simulink model "final"  (R2023b)
settings: Solver=FixedStepAuto  StartTime=0.0  StopTime=60  RelTol=1e-3
undefined symbols (not defined in the file or in its folder): DiscIntNeverNeededParam
libraries: arduinolib x16, simulink x12, mobileRoboticsTrainingLib x1
settings Model: ExtModeTrigDuration=2  Creator=cameronclark  LastModifiedBy=cameronclark
settings OptimizationCC: EnhancedBackFolding=on  PassReuseOutputArgsAs=Individual arguments  ZeroExternalMemoryAtStartup=off  ZeroInternalMemoryAtStartup=off  MaxStackSize=64  OptimizeBlockOrder=speed  DifferentSizesBufferReuse=on  OptimizationCustomize=off  EfficientTunableParamExpr=on
settings DebuggingCC: ParameterTunabilityLossMsg=error
settings HardwareCC: ProdBitPerPointer=32  ProdBitPerSizeT=32  ProdBitPerPtrDiffT=32  ProdLargestAtomicInteger=Long  ProdLargestAtomicFloat=Double  ProdWordSize=32  ProdHWDeviceType=ARM Compatible->ARM Cortex  UseEmbeddedCoderFeatures=off  UseSimulinkCoderFeatures=off
settings SFSimCC: MATLABDynamicMemAlloc=off
settings RTWCC: Description=Embedded Coder  SystemTargetFile=ert.tlc  HardwareBoard=Arduino Nano 33 IoT  TemplateMakefile=ert_default_tmf  Toolchain=Arduino ARM  BuildConfiguration=Faster Runs
settings CodeAppCC: ForceParamTrailComments=on  IgnoreCustomStorageClasses=off  OperatorAnnotations=on  SimulinkDataObjDesc=on  SFDataObjDesc=on  InsertBlockDesc=on
settings ERTTargetCC: SupportContinuousTime=on  SupportNonInlinedSFcns=on  SupportVariableSizeSignals=on  ExtModeTransport=3  ExtModeStaticAlloc=on  ExtModeAutomaticAllocSize=off  ExtModeStaticAllocSize=8192  ExtModeMexFile=ext_xcp  ExtModeIntrfLevel=Level2 - Open

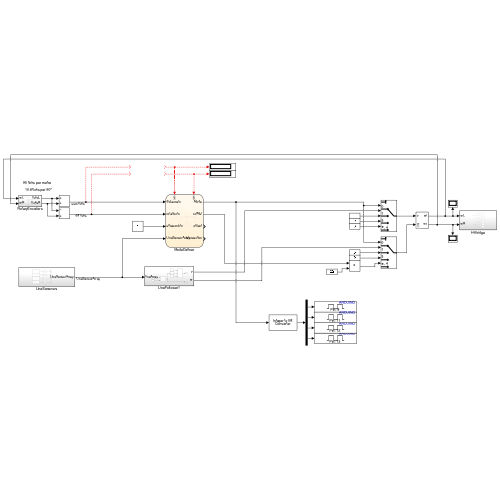
[thumbnail: Simulink's stored preview of the top-level diagram]
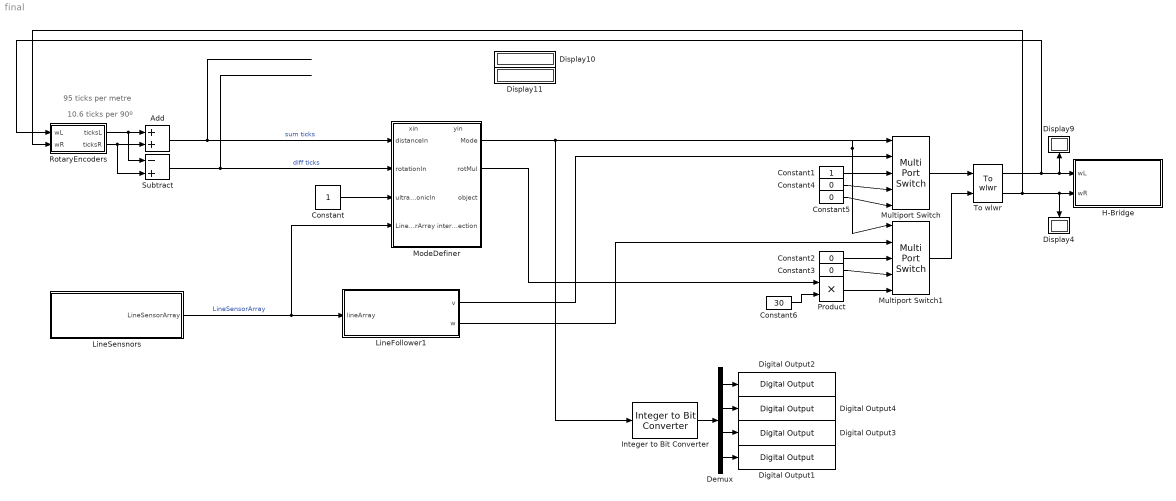
== system final ==
  note: 95 ticks per metre
  note: 10.6 ticks per 90º
  Add : Sum
  Constant : Constant
  Constant1 : Constant
  Constant{2..5} (4 alike) : Constant  Value=0
  Constant6 : Constant  Value=30
  Demux : Demux
  Digital Output1 : arduinolib/Digital Output  pinNumber=13  Direction=output  blockPlatform=arduino
  Digital Output2 : arduinolib/Digital Output  pinNumber=8  Direction=output  blockPlatform=arduino
  Digital Output3 : arduinolib/Digital Output  pinNumber=12  Direction=output  blockPlatform=arduino
  Digital Output4 : arduinolib/Digital Output  pinNumber=11  Direction=output  blockPlatform=arduino
  Display{4,9..11} (4 alike) : Display
  H-Bridge : Subsystem
  Integer to Bit Converter : simulink/Logic and Bit Operations/Integer to Bit Converter  nbits=4  signedInputValues=Unsigned  bitOrder=MSB first  outDtype=Inherit via internal rule
  LineFollower1 : Subsystem
  LineSensnors : Subsystem
  ModeDefiner : Stateflow chart  TreatAsAtomicUnit=on
      settings: PortSchema="{\"entries\":[{\"content\":{\"sides\":[{\"content\":{\"connectorIds\":[\"In4\",\"In5\",\"In3\",\"In6\"]},\"type\":\"ConnectorPlacement.EquallySpacedRectSide\",\"uuid\":\"2e12269d-ccd1-4e68-8415-629d2e368e6d\"},{\"content\":{\"connectorIds\":[\"Out1\",\"Out2\",\"Out3\",\"Out4\"],\"side\":\"RIGHT\"},\"type\":\"ConnectorPlacement.EquallySpacedRectSide\",\"uuid\":\"1564c0f6-61d7-475f-9f3f-a1f2c1915817\"},{\"content\":{\"connectorIds\":[\"In1\",\"In2\"],\"side\":\"TOP\"},\"type\":\"ConnectorPlacement.EquallySpacedRectSide\",\"uuid\":\"729d5d21-cc85-429f-97c7-0630790832c8\"}]},\"type\":\"ConnectorPlacement.EquallySpacedConnector\",\"uuid\":\"65fad4a7-698e-4a16-b156-07c77b4027bb\"}],\"packageUris\":[\"http://schema.mathworks.com/mf0/Connector/R2020b\"],\"version\":\"1.0\"}"
  Multiport Switch : MultiPortSwitch  DataPortOrder=Specify indices  Inputs=5  DataPortIndices={0,1,3,4}  SaturateOnIntegerOverflow=off
  Multiport Switch1 : MultiPortSwitch  DataPortOrder=Specify indices  Inputs=5  DataPortIndices={0,1,3,4}  SaturateOnIntegerOverflow=off  InputSameDT=off
  Product : Product
  RotaryEncoders : Subsystem
  Subtract : Sum  Inputs=-+
  To wlwr : mobileRoboticsTrainingLib/To wlwr  axleLength=0.1  wheelR=0.05
      link override change parameters: Gain=[1 -axleLength/2;1 axleLength/2]
  wires:
  ? -> ModeDefiner/2(yin), Display11/1
  To wlwr/2 -> RotaryEncoders/2(wR), H-Bridge/2(wR), Display4/1
  Subtract/1 -> ModeDefiner/5(rotationIn)  "diff ticks"
  RotaryEncoders/2(ticksR) -> Subtract/2, Add/2
  LineSensnors/1(LineSensorArray) -> ModeDefiner/6(LineSensorArray), LineFollower1/1(lineArray)  "LineSensorArray"
  To wlwr/1 -> RotaryEncoders/1(wL), H-Bridge/1(wL), Display9/1
  Constant/1 -> ModeDefiner/3(ultrasonicIn)
  ? -> ModeDefiner/1(xin), Display10/1
  Add/1 -> ModeDefiner/4(distanceIn)  "sum ticks"
  RotaryEncoders/1(ticksL) -> Subtract/1, Add/1
  Multiport Switch/1 -> To wlwr/1
  Multiport Switch1/1 -> To wlwr/2
  LineFollower1/1(v) -> Multiport Switch/2
  LineFollower1/2(w) -> Multiport Switch1/2
  ModeDefiner/1(Mode) -> Multiport Switch1/1, Multiport Switch/1, Integer to Bit Converter/1
  Constant1/1 -> Multiport Switch/3
  Constant2/1 -> Multiport Switch1/3
  Constant5/1 -> Multiport Switch/5
  Product/1 -> Multiport Switch1/5
  Constant6/1 -> Product/2
  ModeDefiner/2(rotMul) -> Product/1
  Constant4/1 -> Multiport Switch/4
  Constant3/1 -> Multiport Switch1/4
  Integer to Bit Converter/1 -> Demux/1
  Demux/1 -> Digital Output2/1
  Demux/2 -> Digital Output4/1
  Demux/3 -> Digital Output3/1
  Demux/4 -> Digital Output1/1

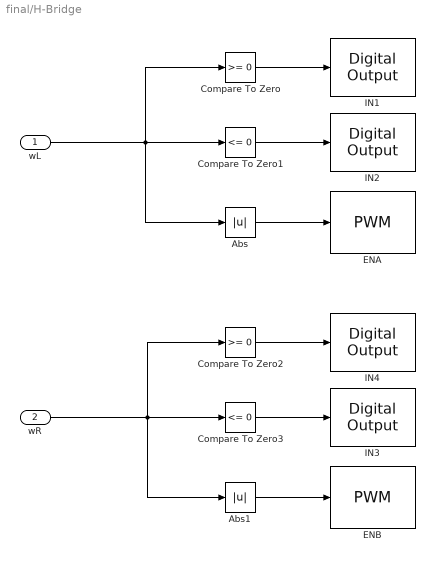
== system final/H-Bridge ==
  wL : Inport
  wR : Inport  Port=2
  Abs : Abs  SaturateOnIntegerOverflow=off
  Abs1 : Abs  SaturateOnIntegerOverflow=off
  Compare To Zero : simulink/Logic and Bit Operations/Compare To Zero  relop=>=  OutDataTypeStr=boolean
  Compare To Zero1 : simulink/Logic and Bit Operations/Compare To Zero  relop=<=  OutDataTypeStr=boolean
  Compare To Zero2 : simulink/Logic and Bit Operations/Compare To Zero  relop=>=  OutDataTypeStr=boolean
  Compare To Zero3 : simulink/Logic and Bit Operations/Compare To Zero  relop=<=  OutDataTypeStr=boolean
  ENA : arduinolib/PWM  pinNumber=2  frequencyType=Default  desiredFrequency=490.2  achievableFrequency=490.2
  ENB : arduinolib/PWM  pinNumber=3  frequencyType=Default  desiredFrequency=490.2  achievableFrequency=490.2
  IN1 : arduinolib/Digital Output  pinNumber=0  Direction=output  blockPlatform=arduino
  IN2 : arduinolib/Digital Output  pinNumber=1  Direction=output  blockPlatform=arduino
  IN3 : arduinolib/Digital Output  pinNumber=5  Direction=output  blockPlatform=arduino
  IN4 : arduinolib/Digital Output  pinNumber=4  Direction=output  blockPlatform=arduino
  wires:
  Compare To Zero1/1 -> IN2/1
  Compare To Zero/1 -> IN1/1
  Abs1/1 -> ENB/1
  Compare To Zero3/1 -> IN3/1
  Compare To Zero2/1 -> IN4/1
  wL/1 -> Compare To Zero/1, Compare To Zero1/1, Abs/1
  Abs/1 -> ENA/1
  wR/1 -> Compare To Zero2/1, Compare To Zero3/1, Abs1/1

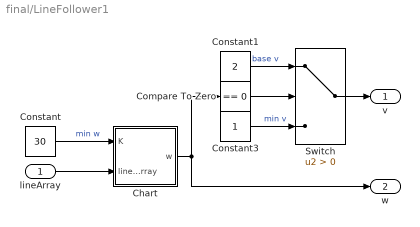
== system final/LineFollower1 ==
  lineArray : Inport
  Chart : Stateflow chart  TreatAsAtomicUnit=on
  Compare To Zero : simulink/Logic and Bit Operations/Compare To Zero  relop===  OutDataTypeStr=boolean
  Constant : Constant  Value=30
  Constant1 : Constant  Value=2
  Constant3 : Constant
  Switch : Switch  Criteria=u2 > Threshold  SaturateOnIntegerOverflow=off  InputSameDT=off
  v : Outport
  w : Outport  Port=2
  wires:
  Constant1/1 -> Switch/1  "base v"
  Chart/1(w) -> Compare To Zero/1, w/1
  Constant3/1 -> Switch/3  "min v"
  Switch/1 -> v/1
  lineArray/1 -> Chart/2(lineArray)
  Compare To Zero/1 -> Switch/2
  Constant/1 -> Chart/1(K)  "min w"

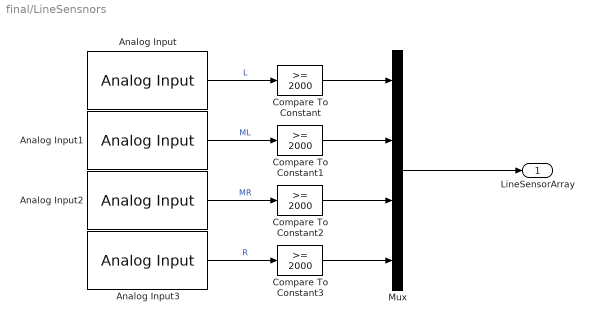
== system final/LineSensnors ==
  Analog Input : arduinolib/Analog Input  pinNumber=7  ReadResultsOnly=off  ConversionTriggerSource=Software  ExternalTriggerType=uint32( 0 )  OutputDataType=uint16  EnableConversionCompleteNotify=off  EnableOuputStatus=off  SampleTime=-1  blockPlatform=arduino
  Analog Input1 : arduinolib/Analog Input  pinNumber=6  ReadResultsOnly=off  ConversionTriggerSource=Software  ExternalTriggerType=uint32( 0 )  OutputDataType=uint16  EnableConversionCompleteNotify=off  EnableOuputStatus=off  SampleTime=-1  blockPlatform=arduino
  Analog Input2 : arduinolib/Analog Input  pinNumber=3  ReadResultsOnly=off  ConversionTriggerSource=Software  ExternalTriggerType=uint32( 0 )  OutputDataType=uint16  EnableConversionCompleteNotify=off  EnableOuputStatus=off  SampleTime=-1  blockPlatform=arduino
  Analog Input3 : arduinolib/Analog Input  pinNumber=2  ReadResultsOnly=off  ConversionTriggerSource=Software  ExternalTriggerType=uint32( 0 )  OutputDataType=uint16  EnableConversionCompleteNotify=off  EnableOuputStatus=off  SampleTime=-1  blockPlatform=arduino
  Compare To Constant{,1..3} (4 alike) : simulink/Logic and Bit Operations/Compare To Constant  relop=>=  const=2000  OutDataTypeStr=boolean
  Mux : Mux
  LineSensorArray : Outport
  wires:
  Mux/1 -> LineSensorArray/1
  Analog Input/1 -> Compare To Constant/1  "L"
  Analog Input1/1 -> Compare To Constant1/1  "ML"
  Analog Input2/1 -> Compare To Constant2/1  "MR"
  Analog Input3/1 -> Compare To Constant3/1  "R"
  Compare To Constant/1 -> Mux/1
  Compare To Constant1/1 -> Mux/2
  Compare To Constant2/1 -> Mux/3
  Compare To Constant3/1 -> Mux/4

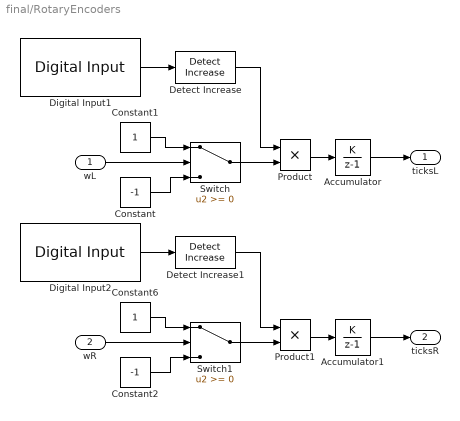
== system final/RotaryEncoders ==
  wL : Inport
  wR : Inport  Port=2
  Accumulator : DiscreteIntegrator  IntegratorMethod=Accumulation: Forward Euler  SampleTime=-1  ICPrevOutput=DiscIntNeverNeededParam  ICPrevScaledInput=DiscIntNeverNeededParam
  Accumulator1 : DiscreteIntegrator  IntegratorMethod=Accumulation: Forward Euler  SampleTime=-1  ICPrevOutput=DiscIntNeverNeededParam  ICPrevScaledInput=DiscIntNeverNeededParam
  Constant : Constant  Value=-1
  Constant1 : Constant
  Constant2 : Constant  Value=-1
  Constant6 : Constant
  Detect Increase : simulink/Logic and Bit Operations/Detect Increase  vinit=0.0  OutDataTypeStr=boolean
  Detect Increase1 : simulink/Logic and Bit Operations/Detect Increase  vinit=0.0  OutDataTypeStr=boolean
  Digital Input1 : arduinolib/Digital Input  pinNumber=9  mode=Default  Direction=input  SampleTime=0.1  blockPlatform=arduino
  Digital Input2 : arduinolib/Digital Input  pinNumber=10  mode=Default  Direction=input  SampleTime=0.1  blockPlatform=arduino
  Product : Product
  Product1 : Product
  Switch : Switch  SaturateOnIntegerOverflow=off  InputSameDT=off
  Switch1 : Switch  SaturateOnIntegerOverflow=off  InputSameDT=off
  ticksL : Outport
  ticksR : Outport  Port=2
  wires:
  wL/1 -> Switch/2
  Constant1/1 -> Switch/1
  Constant/1 -> Switch/3
  Digital Input1/1 -> Detect Increase/1
  Switch/1 -> Product/2
  Accumulator/1 -> ticksL/1
  wR/1 -> Switch1/2
  Constant6/1 -> Switch1/1
  Constant2/1 -> Switch1/3
  Accumulator1/1 -> ticksR/1
  Switch1/1 -> Product1/2
  Product/1 -> Accumulator/1
  Detect Increase/1 -> Product/1
  Detect Increase1/1 -> Product1/1
  Digital Input2/1 -> Detect Increase1/1
  Product1/1 -> Accumulator1/1

== stateflow chart final/ModeDefiner ==
  state Start
    entry:
    Mode = 0; %Drive
    intersections = -1 * ones(5,3,4) %[x y;angle1-4;visited1-4]
    intersection = 1; %the last index of the intersections array
    currentIntersection = 1; %the intersection the robot is at
    objects = -1 * ones(5, 4); %[x y distance rotation]
    object = 1; %last index of the objects array
    stopZoneFound = 0;
    defaultPath=2 %the path to take if there are no unexplored paths on current intersection
  state RotateBackToLine
    entry:
    Mode = 4;
    rotMul = rotMul * -1;
    exit:
    Mode = 0;
  state Explore
    %Go forth and find the next thing
  state DriveAwayFromInterrupt
    entry:
    Mode = 0;
    distanceTarget = distanceIn + 8;
  state RotateToLine
    entry:
    if (LineSensorArray(1) == 0)
    rotMul = 1;
    else
    rotMul = -1;
    end
    Mode = 4;
  state TurnAround
    entry:
    Mode = 4;
    rotationTarget = rotationIn + 21;
    rotMul = 1;
  state RecordObject
    entry:
    objects(object,:) = [xin yin ultrasonicIn rotationIn];
    object = object + 1;
  state DriveBackToLine
    entry:
    Mode = 0;
    distanceTarget = distanceIn + 12
  state CentreOnIntersection
    entry:
    %rot mul determines the direction of the rotation
    if (LineSensorArray(1) == 0)
    rotMul = 1;
    else
    rotMul = -1;
    end
    distanceTarget = distanceIn + 12;
    Mode = 0;
  state SenseNewIntersection
    entry:
    Mode = 4; % rotate
    if all(LineSensorArray(2:3)==0) %is there an intersection infront
    rotationTarget = 0; %assume that robot is at an intersection
    else
    %the robot might be just off the line, so if it has to rotate less than 45° to find a line
    %return to the path
    rotationTarget = rotationIn + 5*rotMul;
    end
    rotationHalf = rotationIn + 21*rotMul; %half rotatation target
    rotationFull = rotationIn + 42*rotMul; %full rotation target
    lineSensorRising = 2.5 - 0.5*rotMul; %the rising edge line sensor
    lineSensorFalling = 2.5 + 0.5*rotMul; %the falling edge line sensor
    %when detecting a line, one sensor will have a rising edge, and one will have a falling edge,
    %take the average of those two angles will give the angle of the intersection
    risingEdge = LineSensorArray(lineSensorRising);
    fallingEdge = LineSensorArray(lineSensorFalling);
    fallingEdgeDetected = 0;
    rotationFalling = 0;
    path = 1;
    if (~LineSensorArray(2) | ~LineSensorArray(3))
    %robot is facing a path to start with
    intersections(intersection,2,path) = rotationIn;
    intersections(intersection,3,path) = 0;
    path = path + 1;
    end
    during:
    if rotationTarget
    if (rotMul*(rotationTarget-rotationIn) >= 0) & all(LineSensorArray(2:3)==0)
    %robot rotated less than 45° and is back on path, thus, no intersection
    Mode = 1;
    end
    end
    if fallingEdge & ~LineSensorArray(lineSensorFalling)
    rotationFalling = rotationIn; %initial side of a path detected
    fallingEdgeDetected = 1;
    end
    if ~risingEdge & LineSensorArray(lineSensorRising)
    if fallingEdgeDetected
    %other side of the intersection
    intersections(intersection,2,path) = (rotationIn + rotationFalling)/2;
    fallingEdgeDetected = 0;
    if rotationHalf & (abs(intersections(intersection,2,path) - rotationHalf) <= 3)
    %180° rotated thus, it is the path we came from, mark as return path.
    intersections(intersection,3,path) = 2 + stopZoneFound;
    rotationHalf = 0;
    else
    %else mark as unexplored
    intersections(intersection,3,path) = 0;
    end
    path = path + 1;
    end
    end
    %updating edges
    risingEdge = LineSensorArray(lineSensorRising);
    fallingEdge = LineSensorArray(lineSensorFalling);
  state Stop
    entry:
    Mode = 3;
  state PickPath
    entry:
    Mode = 4;
    if stopZoneFound %stop zone found so mark path that returns to stop zone
    if ~any(intersections(currentIntersection,3,:)==3)
    for path = 1:4
    if abs(abs(mod(intersections(currentIntersection,2,path)-rotationIn,42))-21) <= 3
    intersections(currentIntersection,3,path) = 3;
    break;
    end
    end
    end
    end
    if any(intersections(currentIntersection,3,:)==0)
    %there is an unexplored path so take it
    for path = 4:-1:1
    if ~intersections(currentIntersection,3,path)
    intersections(currentIntersection,3,path) = 1;
    rotationTarget = intersections(currentIntersection,2,path)
    if rotationTarget-rotationIn > 0
    rotMul = 1;
    else
    rotMul = -1;
    end
    break;
    end
    end
    else
    %go back down return path OR stop zone path if no unexplored paths left
    for path = 1:4
    if intersections(currentIntersection,3,path)==defaultPath
    rotationTarget = intersections(currentIntersection,2,path)
    if rotationTarget-rotationIn > 0
    rotMul = 1;
    else
    rotMul = -1;
    end
    break
    end
    end
    end
  state CheckForOldIntersection
    entry:
    %checks if the x y of the robot match any x y of any recorded intersections
    oldIntersection = 0;
    for currentIntersection = 1:5
    if ~all(intersections(currentIntersection,3,:)==-1)
    if abs(intersections(currentIntersection,1,1)-xin) <= 9
    if abs(intersections(currentIntersection,1,2)-yin) <= 9
    oldIntersection = 1;
    break;
    end
    end
    end
    end
  state AddIntersection
    entry:
    %next intersection in array
    intersections(intersection,1,1) = xin;
    intersections(intersection,1, 2) = yin;
    currentIntersection = intersection;
    intersection = intersection + 1;
  (default) -> Start
  Start -> Explore
  RotateBackToLine -> Explore : [all(LineSensorArray(2:3)==0)]
  DriveBackToLine -> RotateBackToLine : [distanceIn>=distanceTarget]
  Explore -> (junction 118) [order 1] : [(LineSensorArray(1) == 0) | (LineSensorArray(4) == 0)]{Mode=3}%interrupt triggered
  DriveAwayFromInterrupt -> Explore : [distanceIn >= distanceTarget]
  Explore -> TurnAround [order 2] : [all(LineSensorArray==1)]
      | %at a dead end
  TurnAround -> DriveAwayFromInterrupt : [rotationIn>rotationTarget]
  RecordObject -> TurnAround
  (junction 118) -> RotateToLine [order 3] : [all(LineSensorArray(2:3)==1)]
      | %Robot is off the line
  (junction 118) -> RecordObject [order 1] : [ultrasonicIn & (ultrasonicIn <= 0.5)]
      | %at measurement line
  (junction 118) -> CentreOnIntersection [order 2] : [(LineSensorArray(1) == 0) & (LineSensorArray(4) == 0)]
      | %At a T intersection
  (junction 118) -> CentreOnIntersection [order 4] : %default: assume at intersection
  PickPath -> DriveAwayFromInterrupt : [rotMul*(rotationTarget-rotationIn) <= 0]
      | %rotated to target path
  RotateToLine -> DriveBackToLine : [all(LineSensorArray(2:3)==0)]
  (junction 99) -> TurnAround [order 1] : [any(any(intersections(:,3,:) == 0))]{stopZoneFound =1;}
      | %There are unexplore paths, return to them
  SenseNewIntersection -> DriveBackToLine [order 1] : [Mode==1]
      | %continue back to path
  CentreOnIntersection -> (junction 93) : [distanceIn >= distanceTarget]
  (junction 93) -> (junction 99) [order 1] : [all(LineSensorArray==0)]
      | %At a stop zone not an intersection
  (junction 93) -> CheckForOldIntersection [order 2] : %default: at intersection
  (junction 99) -> Stop [order 2] : %All paths explored
  CheckForOldIntersection -> SenseNewIntersection [order 1] : [~oldIntersection]
  (junction 113) -> PickPath [order 1] : [any(any(intersections(:,3,:)==0))]{defaultPath=2;}
      | %there are still unexplored intersections
      | %thus, go down the return intersections
  CheckForOldIntersection -> (junction 113) [order 2] : [oldIntersection]
      | %this intersection has been found
  (junction 113) -> PickPath [order 2] : {defaultPath=3;}
      | %there are no unexplored intersections
      | %thus, return to stop zone
  AddIntersection -> PickPath
  SenseNewIntersection -> AddIntersection [order 2] : [(abs(rotationIn - rotationFull) <= 2)]{defaultPath==2}
      | %fully rotated so intersection recorded
  data: xin input; yin input; ultrasonicIn input; Mode output =0; rotMul output; distanceIn input; distanceTarget local; rotationIn input; LineSensorArray input; fallingEdge local; rotationHalf local; rotationFull local; path local; rotationTarget local; risingEdge local; lineSensorFalling local; lineSensorRising local; rotationFalling local; fallingEdgeDetected local; intersections local; oldIntersection local; currentIntersection local; stopZoneFound local; defaultPath local; objects local; object output; intersection output

== stateflow chart final/LineFollower1/Chart ==
  state ComputeW
    %code for the line array
    during:
    w = K*(lineArray(3)-lineArray(2));
  (default) -> ComputeW
  data: w output; K input; lineArray input
